simulink model "mInterpolatedStateSpaceThermalModel_TwoCoolSys"  (R2021b)
settings: Solver=VariableStepAuto  StartTime=0.0  StopTime=4000  FixedStep=0.2  RelTol=1e-3  AbsTol=1e-3
values from neighbouring files (symbols this model uses):
  TnodesInit = [TcoolantIn;330;290]    [tInterpolatedStateSpaceThermalModel.m]
libraries: mcadROM_lib x1
settings Model: Creator=agonzale  LastModifiedBy=agonzale
settings SolverCC: AutoScaleAbsTol=off  NumberNewtonIterations=3

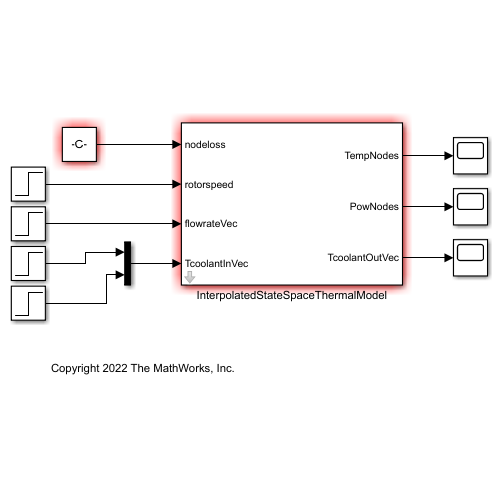
[thumbnail: Simulink's stored preview of the top-level diagram]
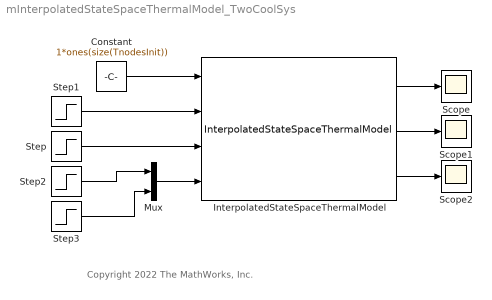
== system mInterpolatedStateSpaceThermalModel_TwoCoolSys ==
  note: Copyright 2022 The MathWorks, Inc.
  Constant : Constant  Value=1*ones(size(TnodesInit))
  InterpolatedStateSpaceThermalModel : mcadROM_lib/InterpolatedStateSpaceThermalModel  BkptsStruct=BkptsStruct  AMatND=AmatND  BMatND=BmatND  ResMatND=ResMatND  CoolAdjMat=AdjacencyMat  CoolantArrayIdxs=[5 25] % dummy value  InletCoolantIdxs=InletCoolIdxs  OutletCoolantIdxs=OutletCoolIdxs  TnodesInit=TnodesInit
  Mux : Mux  Inputs=2
  Scope : Scope
  Scope1 : Scope
  Scope2 : Scope
  Step : Step  Time=1500  Before=[5,6]  After=[9,10]  SampleTime=0
  Step1 : Step  Time=2500  Before=1000  After=4000  SampleTime=0
  Step2 : Step  Time=1000  Before=25  After=30  SampleTime=0
  Step3 : Step  Time=3000  Before=35  After=45  SampleTime=0
  wires:
  Constant/1 -> InterpolatedStateSpaceThermalModel/1
  Step1/1 -> InterpolatedStateSpaceThermalModel/2
  Step/1 -> InterpolatedStateSpaceThermalModel/3
  InterpolatedStateSpaceThermalModel/1 -> Scope/1
  InterpolatedStateSpaceThermalModel/2 -> Scope1/1
  InterpolatedStateSpaceThermalModel/3 -> Scope2/1
  Mux/1 -> InterpolatedStateSpaceThermalModel/4
  Step2/1 -> Mux/1
  Step3/1 -> Mux/2
